simulink model "KD2BD_Pacsat_Modem"  (R2013a)
settings: Solver=ode45  StartTime=0.0  StopTime=3  RelTol=1e-3
libraries: dsparch4 x2, commchan3 x1, commrandsrc2 x1, commutil2 x1, simulink_extras x1
settings Model: Creator=tibbs2010  LastModifiedBy=tibbs2010

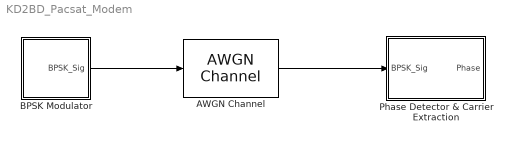
== system KD2BD_Pacsat_Modem ==
  AWGN Channel : commchan3/AWGN Channel  InputProcessing=Columns as channels (frame based)  seed=67  noiseMode="Signal to noise ratio  (SNR)"  EbNodB=10  EsNodB=10  SNRdB=.5  bitsPerSym=1  Ps=1  Tsym=1  variance=1
  BPSK Modulator : Subsystem
  Phase Detector & Carrier Extraction : Subsystem
  wires:
  BPSK Modulator/1(BPSK_Sig) -> AWGN Channel/1
  AWGN Channel/1 -> Phase Detector & Carrier Extraction/1(BPSK_Sig)

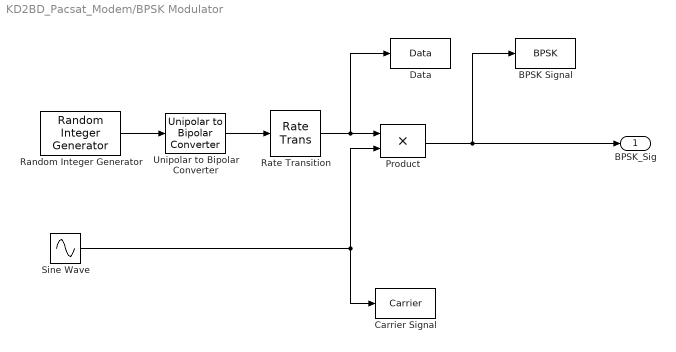
== system KD2BD_Pacsat_Modem/BPSK Modulator ==
  BPSK Signal : ToWorkspace  VariableName=BPSK  SampleTime=-1  SaveFormat=Timeseries
  Carrier Signal : ToWorkspace  VariableName=Carrier  SampleTime=-1  SaveFormat=Timeseries
  Data : ToWorkspace  VariableName=Data  SampleTime=-1  SaveFormat=Timeseries
  Product : Product  SaturateOnIntegerOverflow=on  OutDataTypeStr=Inherit: Same as first input
  Random Integer Generator : commrandsrc2/Random Integer Generator  mul=2  seed=randseed  Ts=1/32  frameBased=off  sampPerFrame=1  orient=off  outDataType=double
  Rate Transition : RateTransition
  Sine Wave : Sin  Frequency=1200*2*pi  Phase=pi/2  SampleTime=1e-5
  Unipolar to Bipolar Converter : commutil2/Unipolar to Bipolar Converter  M=2  polarity=Positive  dataType=Same as input
  BPSK_Sig : Outport
  wires:
  Random Integer Generator/1 -> Unipolar to Bipolar Converter/1
  Rate Transition/1 -> Data/1, Product/1
  Sine Wave/1 -> Carrier Signal/1, Product/2
  Product/1 -> BPSK Signal/1, BPSK_Sig/1
  Unipolar to Bipolar Converter/1 -> Rate Transition/1

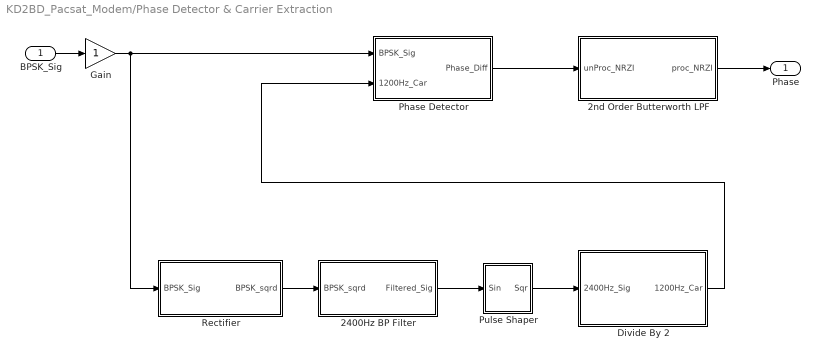
== system KD2BD_Pacsat_Modem/Phase Detector & Carrier Extraction ==
  BPSK_Sig : Inport
  2400Hz BP Filter : Subsystem
  "2nd Order Butterworth LPF " : Subsystem
  Divide By 2 : Subsystem
  Gain : Gain
  Phase Detector : Subsystem
  Pulse Shaper : Subsystem
  Rectifier : Subsystem
  Phase : Outport
  wires:
  BPSK_Sig/1 -> Gain/1
  Rectifier/1(BPSK_sqrd) -> 2400Hz BP Filter/1(BPSK_sqrd)
  Pulse Shaper/1(Sqr) -> Divide By 2/1(2400Hz_Sig)
  Gain/1 -> Phase Detector/1(BPSK_Sig), Rectifier/1(BPSK_Sig)
  Divide By 2/1(1200Hz_Car) -> Phase Detector/2(1200Hz_Car)
  2400Hz BP Filter/1(Filtered_Sig) -> Pulse Shaper/1(Sin)
  Phase Detector/1(Phase_Diff) -> "2nd Order Butterworth LPF "/1(unProc_NRZI)
  "2nd Order Butterworth LPF "/1(proc_NRZI) -> Phase/1

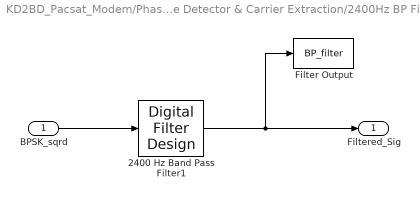
== system KD2BD_Pacsat_Modem/Phase Detector & Carrier Extraction/2400Hz BP Filter ==
  BPSK_sqrd : Inport
  2400 Hz Band Pass Filter1 : dsparch4/Digital Filter Design  mwdsp_browser_bugfix_var=off
  Filter Output : ToWorkspace  VariableName=BP_filter  SampleTime=-1  SaveFormat=Timeseries
  Filtered_Sig : Outport
  wires:
  2400 Hz Band Pass Filter1/1 -> Filter Output/1, Filtered_Sig/1
  BPSK_sqrd/1 -> 2400 Hz Band Pass Filter1/1

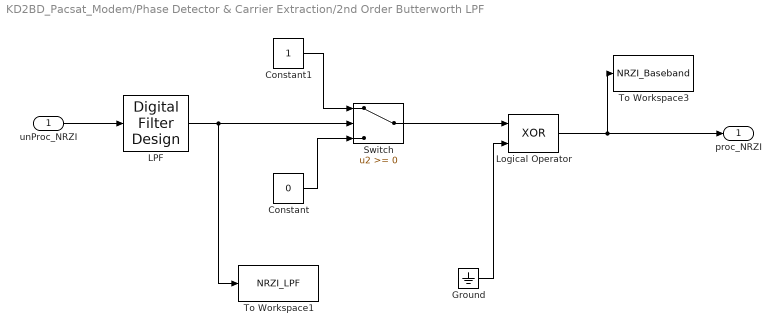
== system KD2BD_Pacsat_Modem/Phase Detector & Carrier Extraction/2nd Order Butterworth LPF  ==
  unProc_NRZI : Inport
  Constant : Constant  Value=0
  Constant1 : Constant
  Ground : Ground
  LPF : dsparch4/Digital Filter Design  mwdsp_browser_bugfix_var=off
  Logical Operator : Logic  Operator=XOR  IconShape=distinctive  AllPortsSameDT=off  OutDataTypeStr=boolean
  Switch : Switch
  To Workspace1 : ToWorkspace  VariableName=NRZI_LPF  SampleTime=-1  SaveFormat=Timeseries
  To Workspace3 : ToWorkspace  VariableName=NRZI_Baseband  SampleTime=-1  SaveFormat=Timeseries
  proc_NRZI : Outport
  wires:
  LPF/1 -> To Workspace1/1, Switch/2
  unProc_NRZI/1 -> LPF/1
  Constant/1 -> Switch/3
  Switch/1 -> Logical Operator/1
  Constant1/1 -> Switch/1
  Ground/1 -> Logical Operator/2
  Logical Operator/1 -> proc_NRZI/1, To Workspace3/1

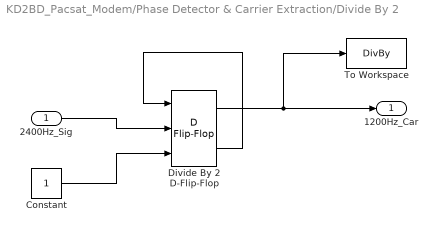
== system KD2BD_Pacsat_Modem/Phase Detector & Carrier Extraction/Divide By 2 ==
  2400Hz_Sig : Inport
  Constant : Constant
  Divide By 2 D-Flip-Flop : simulink_extras/Flip Flops/D Flip-Flop
  To Workspace : ToWorkspace  VariableName=DivBy  SampleTime=-1  SaveFormat=Timeseries
  1200Hz_Car : Outport
  wires:
  Divide By 2 D-Flip-Flop/2 -> Divide By 2 D-Flip-Flop/1
  2400Hz_Sig/1 -> Divide By 2 D-Flip-Flop/2
  Divide By 2 D-Flip-Flop/1 -> 1200Hz_Car/1, To Workspace/1
  Constant/1 -> Divide By 2 D-Flip-Flop/3

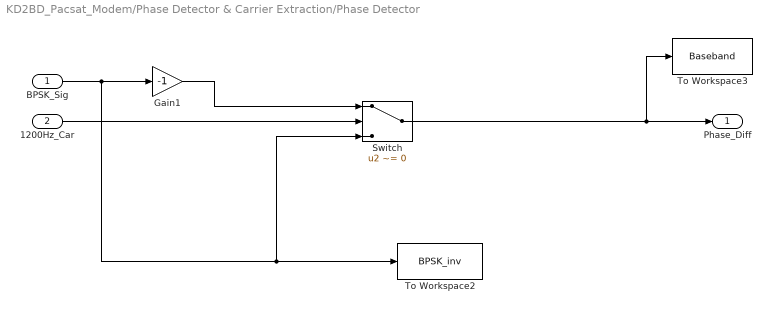
== system KD2BD_Pacsat_Modem/Phase Detector & Carrier Extraction/Phase Detector ==
  BPSK_Sig : Inport
  1200Hz_Car : Inport  Port=2
  Gain1 : Gain  Gain=-1
  Switch : Switch  Criteria=u2 ~= 0
  To Workspace2 : ToWorkspace  VariableName=BPSK_inv  SampleTime=-1  SaveFormat=Timeseries
  To Workspace3 : ToWorkspace  VariableName=Baseband  SampleTime=-1  SaveFormat=Timeseries
  Phase_Diff : Outport
  wires:
  1200Hz_Car/1 -> Switch/2
  BPSK_Sig/1 -> To Workspace2/1, Switch/3, Gain1/1
  Switch/1 -> To Workspace3/1, Phase_Diff/1
  Gain1/1 -> Switch/1

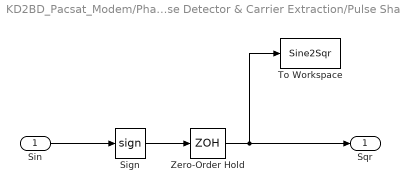
== system KD2BD_Pacsat_Modem/Phase Detector & Carrier Extraction/Pulse Shaper ==
  Sin : Inport
  Sign : Signum
  To Workspace : ToWorkspace  VariableName=Sine2Sqr  SampleTime=-1  SaveFormat=Timeseries
  Zero-Order Hold : ZeroOrderHold  SampleTime=-1
  Sqr : Outport
  wires:
  Zero-Order Hold/1 -> To Workspace/1, Sqr/1
  Sign/1 -> Zero-Order Hold/1
  Sin/1 -> Sign/1

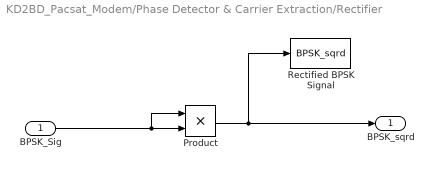
== system KD2BD_Pacsat_Modem/Phase Detector & Carrier Extraction/Rectifier ==
  BPSK_Sig : Inport
  Product : Product
  Rectified BPSK Signal : ToWorkspace  VariableName=BPSK_sqrd  SampleTime=-1  SaveFormat=Timeseries
  BPSK_sqrd : Outport
  wires:
  BPSK_Sig/1 -> Product/1, Product/2
  Product/1 -> Rectified BPSK Signal/1, BPSK_sqrd/1
